simulink model "final"  (R2024a)
settings: Solver=ode23t  StartTime=0.0  StopTime=1  RelTol=1e-6
model workspace (MAT data in the model file):
  Ts = 0.10201388834
undefined symbols (not defined in the file or in its folder): DiscIntNeverNeededParam, Ion, Lithium
libraries: spsIGBTDiodeLib x13, slpidlib x9, spsSeriesRLCBranchLib x7, spsCurrentMeasurementLib x6, spsThreePhaseSeriesRLCBranchLib x6, spsThreePhaseVIMeasurementLib x5, spsAlphaBetaZerotodq0Lib x4, spsGroundLib x3, spsPower3phInstantaneousLib x3, spsMosfetLib x2, simulink x2, spsdq0toabcLib x2
(part 2 of 3)

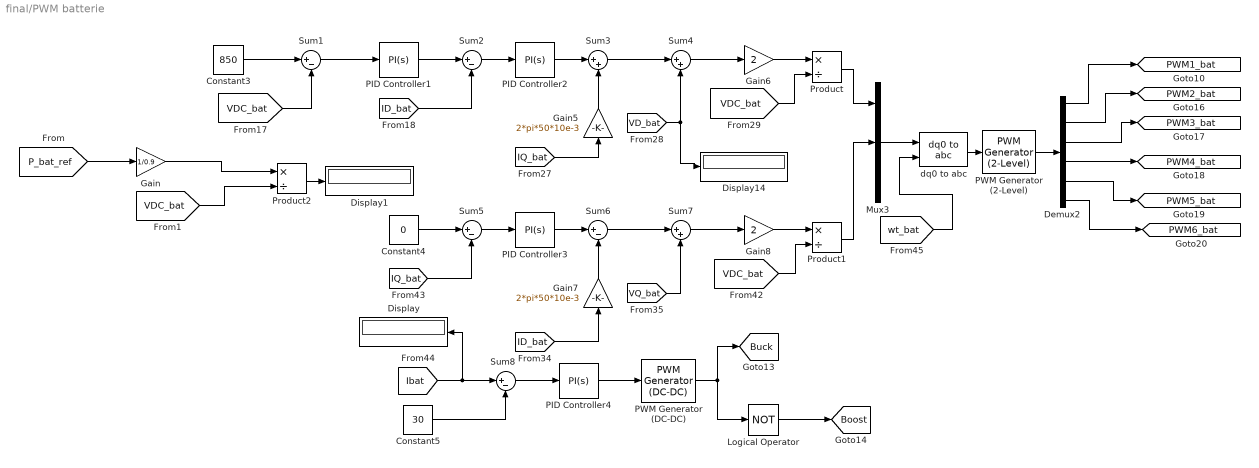
== system final/PWM batterie ==
  Constant3 : Constant  Value=850
  Constant4 : Constant  Value=0
  Constant5 : Constant  Value=30
  Demux2 : Demux  Outputs=6
  Display : Display
  Display1 : Display
  Display14 : Display
  Gain : Gain  Gain=1/0.9
  Gain5 : Gain  Gain=2*pi*50*10e-3
  Gain6 : Gain  Gain=2
  Gain7 : Gain  Gain=2*pi*50*10e-3
  Gain8 : Gain  Gain=2
  Logical Operator : Logic  Operator=NOT  AllPortsSameDT=off  OutDataTypeStr=boolean
  Mux3 : Mux  Inputs=3
  PID Controller1 : slpidlib/PID Controller  Controller=PI  Form=Parallel  TimeDomain=Continuous-time  UseExternalTs=off  SampleTime=-1  IntegratorMethod=Forward Euler  FilterMethod=Forward Euler  ControllerParametersSource=internal  P=0.5  I=5  UseKiTs=off  D=0  UseExternalDerivativeSource=off  N=100  UseFilter=on  TunerSelectOption=Transfer Function Based (PID Tuner App)  InitialConditionSource=internal  InitialConditionForIntegrator=0  InitialConditionForFilter=0  DifferentiatorICPrevScaledInput=0  ExternalReset=none  TrackingMode=off  Kt=1  LimitOutput=off  SatLimitsSource=internal  UpperSaturationLimit=inf  LowerSaturationLimit=-inf  LinearizeAsGain=on  AntiWindupMode=none  Kb=1  LimitIntegrator=off  UpperIntegratorSaturationLimit=inf  LowerIntegratorSaturationLimit=-inf  POutMin=[]  POutMax=[]  IOutMin=[]  IOutMax=[]  DOutMin=[]  DOutMax=[]  NOutMin=[]  NOutMax=[]  SumOutMin=[]  SumOutMax=[]  SaturationOutMin=[]  SaturationOutMax=[]  PParamMin=[]  PParamMax=[]  IParamMin=[]  IParamMax=[]  DParamMin=[]  DParamMax=[]  NParamMin=[]  NParamMax=[]  KbParamMin=[]  KbParamMax=[]  KtParamMin=[]  KtParamMax=[]  KbOutMin=[]  KbOutMax=[]  KtOutMin=[]  KtOutMax=[]  IntegratorOutMin=[]  IntegratorOutMax=[]  FilterOutMin=[]  FilterOutMax=[]  SumI1OutMin=[]  SumI1OutMax=[]  SumI2OutMin=[]  SumI2OutMax=[]  SumI3OutMin=[]  SumI3OutMax=[]  SumI4OutMin=[]  SumI4OutMax=[]  SumDOutMin=[]  SumDOutMax=[]  DifferentiatorOutMin=[]  DifferentiatorOutMax=[]  FilterDiffOutCoefMin=[]  FilterDiffOutCoefMax=[]  ReciprocalOutMin=[]  ReciprocalOutMax=[]  SumDenOutMin=[]  SumDenOutMax=[]  SumNumOutMin=[]  SumNumOutMax=[]  DivideOutMin=[]  DivideOutMax=[]  UdiffTsProdOutMin=[]  UdiffTsProdOutMax=[]  NTsProdOutMin=[]  NTsProdOutMax=[]  UintegralTsProdOutMin=[]  UintegralTsProdOutMax=[]  UngainTsProdOutMin=[]  UngainTsProdOutMax=[]  ClampingZeroOutDataTypeStr=Inherit: Inherit via back propagation  ClampingZeroOutMin=[]  ClampingZeroOutMax=[]  FilterDenConstantOutDataTypeStr=Inherit: Inherit via back propagation  FilterDenConstantOutMin=[]  FilterDenConstantOutMax=[]  PCopyOutDataTypeStr=Inherit: Inherit via back propagation  PCopyOutMin=[]  PCopyOutMax=[]  NCopyOutDataTypeStr=Inherit: Inherit via back propagation  NCopyOutMin=[]  NCopyOutMax=[]  IntegratorContinuousStateAttributes=''  IntegratorStateMustResolveToSignalObject=off  IntegratorRTWStateStorageClass=Auto  FilterContinuousStateAttributes=''  FilterStateMustResolveToSignalObject=off  FilterRTWStateStorageClass=Auto  ParallelPVariant=InternalParameters  IdealPVariant=Disabled  IVariant=InternalParameters  DVariant=Disabled  IntegratorVariant=Continuous  SatVariant=Disabled  AWVariant=Passthrough  PCopyVariant=Disabled  TRVariant=Disabled  FdbkBlocksVariant=Forward  IdealPFdbkVariant=Disabled  SatFdbkVariant=Disabled  DerivativeFilterVariant=Disabled  NVariant=Disabled  NCopyVariant=Disabled_SignalSpec  FilterICVariant=Disabled  IntegratorICVariant=InternalICs  ExternalResetVariant=Disabled  TRSumVariant=Passthrough  SumFdbkVariant=Disabled  SumVariant=Sum_PI  TsampFilterVariant=InternalTs  TsampNgainVariant=Passthrough  TsampIntegralVariant=Disabled_SignalSpec  ExternalSaturationOutDataTypeStr=Inherit: Same as second input  DerivativeSourceVariant=Disabled
  PID Controller2 : slpidlib/PID Controller  Controller=PI  Form=Parallel  TimeDomain=Continuous-time  UseExternalTs=off  SampleTime=-1  IntegratorMethod=Forward Euler  FilterMethod=Forward Euler  ControllerParametersSource=internal  P=25  I=500  UseKiTs=off  D=0  UseExternalDerivativeSource=off  N=100  UseFilter=on  TunerSelectOption=Transfer Function Based (PID Tuner App)  InitialConditionSource=internal  InitialConditionForIntegrator=0  InitialConditionForFilter=0  DifferentiatorICPrevScaledInput=0  ExternalReset=none  TrackingMode=off  Kt=1  LimitOutput=off  SatLimitsSource=internal  UpperSaturationLimit=inf  LowerSaturationLimit=-inf  LinearizeAsGain=on  AntiWindupMode=none  Kb=1  LimitIntegrator=off  UpperIntegratorSaturationLimit=inf  LowerIntegratorSaturationLimit=-inf  POutMin=[]  POutMax=[]  IOutMin=[]  IOutMax=[]  DOutMin=[]  DOutMax=[]  NOutMin=[]  NOutMax=[]  SumOutMin=[]  SumOutMax=[]  SaturationOutMin=[]  SaturationOutMax=[]  PParamMin=[]  PParamMax=[]  IParamMin=[]  IParamMax=[]  DParamMin=[]  DParamMax=[]  NParamMin=[]  NParamMax=[]  KbParamMin=[]  KbParamMax=[]  KtParamMin=[]  KtParamMax=[]  KbOutMin=[]  KbOutMax=[]  KtOutMin=[]  KtOutMax=[]  IntegratorOutMin=[]  IntegratorOutMax=[]  FilterOutMin=[]  FilterOutMax=[]  SumI1OutMin=[]  SumI1OutMax=[]  SumI2OutMin=[]  SumI2OutMax=[]  SumI3OutMin=[]  SumI3OutMax=[]  SumI4OutMin=[]  SumI4OutMax=[]  SumDOutMin=[]  SumDOutMax=[]  DifferentiatorOutMin=[]  DifferentiatorOutMax=[]  FilterDiffOutCoefMin=[]  FilterDiffOutCoefMax=[]  ReciprocalOutMin=[]  ReciprocalOutMax=[]  SumDenOutMin=[]  SumDenOutMax=[]  SumNumOutMin=[]  SumNumOutMax=[]  DivideOutMin=[]  DivideOutMax=[]  UdiffTsProdOutMin=[]  UdiffTsProdOutMax=[]  NTsProdOutMin=[]  NTsProdOutMax=[]  UintegralTsProdOutMin=[]  UintegralTsProdOutMax=[]  UngainTsProdOutMin=[]  UngainTsProdOutMax=[]  ClampingZeroOutDataTypeStr=Inherit: Inherit via back propagation  ClampingZeroOutMin=[]  ClampingZeroOutMax=[]  FilterDenConstantOutDataTypeStr=Inherit: Inherit via back propagation  FilterDenConstantOutMin=[]  FilterDenConstantOutMax=[]  PCopyOutDataTypeStr=Inherit: Inherit via back propagation  PCopyOutMin=[]  PCopyOutMax=[]  NCopyOutDataTypeStr=Inherit: Inherit via back propagation  NCopyOutMin=[]  NCopyOutMax=[]  IntegratorContinuousStateAttributes=''  IntegratorStateMustResolveToSignalObject=off  IntegratorRTWStateStorageClass=Auto  FilterContinuousStateAttributes=''  FilterStateMustResolveToSignalObject=off  FilterRTWStateStorageClass=Auto  ParallelPVariant=InternalParameters  IdealPVariant=Disabled  IVariant=InternalParameters  DVariant=Disabled  IntegratorVariant=Continuous  SatVariant=Disabled  AWVariant=Passthrough  PCopyVariant=Disabled  TRVariant=Disabled  FdbkBlocksVariant=Forward  IdealPFdbkVariant=Disabled  SatFdbkVariant=Disabled  DerivativeFilterVariant=Disabled  NVariant=Disabled  NCopyVariant=Disabled_SignalSpec  FilterICVariant=Disabled  IntegratorICVariant=InternalICs  ExternalResetVariant=Disabled  TRSumVariant=Passthrough  SumFdbkVariant=Disabled  SumVariant=Sum_PI  TsampFilterVariant=InternalTs  TsampNgainVariant=Passthrough  TsampIntegralVariant=Disabled_SignalSpec  ExternalSaturationOutDataTypeStr=Inherit: Same as second input  DerivativeSourceVariant=Disabled
  PID Controller3 : slpidlib/PID Controller  Controller=PI  Form=Parallel  TimeDomain=Continuous-time  UseExternalTs=off  SampleTime=-1  IntegratorMethod=Forward Euler  FilterMethod=Forward Euler  ControllerParametersSource=internal  P=25  I=500  UseKiTs=off  D=0  UseExternalDerivativeSource=off  N=100  UseFilter=on  TunerSelectOption=Transfer Function Based (PID Tuner App)  InitialConditionSource=internal  InitialConditionForIntegrator=0  InitialConditionForFilter=0  DifferentiatorICPrevScaledInput=0  ExternalReset=none  TrackingMode=off  Kt=1  LimitOutput=off  SatLimitsSource=internal  UpperSaturationLimit=inf  LowerSaturationLimit=-inf  LinearizeAsGain=on  AntiWindupMode=none  Kb=1  LimitIntegrator=off  UpperIntegratorSaturationLimit=inf  LowerIntegratorSaturationLimit=-inf  POutMin=[]  POutMax=[]  IOutMin=[]  IOutMax=[]  DOutMin=[]  DOutMax=[]  NOutMin=[]  NOutMax=[]  SumOutMin=[]  SumOutMax=[]  SaturationOutMin=[]  SaturationOutMax=[]  PParamMin=[]  PParamMax=[]  IParamMin=[]  IParamMax=[]  DParamMin=[]  DParamMax=[]  NParamMin=[]  NParamMax=[]  KbParamMin=[]  KbParamMax=[]  KtParamMin=[]  KtParamMax=[]  KbOutMin=[]  KbOutMax=[]  KtOutMin=[]  KtOutMax=[]  IntegratorOutMin=[]  IntegratorOutMax=[]  FilterOutMin=[]  FilterOutMax=[]  SumI1OutMin=[]  SumI1OutMax=[]  SumI2OutMin=[]  SumI2OutMax=[]  SumI3OutMin=[]  SumI3OutMax=[]  SumI4OutMin=[]  SumI4OutMax=[]  SumDOutMin=[]  SumDOutMax=[]  DifferentiatorOutMin=[]  DifferentiatorOutMax=[]  FilterDiffOutCoefMin=[]  FilterDiffOutCoefMax=[]  ReciprocalOutMin=[]  ReciprocalOutMax=[]  SumDenOutMin=[]  SumDenOutMax=[]  SumNumOutMin=[]  SumNumOutMax=[]  DivideOutMin=[]  DivideOutMax=[]  UdiffTsProdOutMin=[]  UdiffTsProdOutMax=[]  NTsProdOutMin=[]  NTsProdOutMax=[]  UintegralTsProdOutMin=[]  UintegralTsProdOutMax=[]  UngainTsProdOutMin=[]  UngainTsProdOutMax=[]  ClampingZeroOutDataTypeStr=Inherit: Inherit via back propagation  ClampingZeroOutMin=[]  ClampingZeroOutMax=[]  FilterDenConstantOutDataTypeStr=Inherit: Inherit via back propagation  FilterDenConstantOutMin=[]  FilterDenConstantOutMax=[]  PCopyOutDataTypeStr=Inherit: Inherit via back propagation  PCopyOutMin=[]  PCopyOutMax=[]  NCopyOutDataTypeStr=Inherit: Inherit via back propagation  NCopyOutMin=[]  NCopyOutMax=[]  IntegratorContinuousStateAttributes=''  IntegratorStateMustResolveToSignalObject=off  IntegratorRTWStateStorageClass=Auto  FilterContinuousStateAttributes=''  FilterStateMustResolveToSignalObject=off  FilterRTWStateStorageClass=Auto  ParallelPVariant=InternalParameters  IdealPVariant=Disabled  IVariant=InternalParameters  DVariant=Disabled  IntegratorVariant=Continuous  SatVariant=Disabled  AWVariant=Passthrough  PCopyVariant=Disabled  TRVariant=Disabled  FdbkBlocksVariant=Forward  IdealPFdbkVariant=Disabled  SatFdbkVariant=Disabled  DerivativeFilterVariant=Disabled  NVariant=Disabled  NCopyVariant=Disabled_SignalSpec  FilterICVariant=Disabled  IntegratorICVariant=InternalICs  ExternalResetVariant=Disabled  TRSumVariant=Passthrough  SumFdbkVariant=Disabled  SumVariant=Sum_PI  TsampFilterVariant=InternalTs  TsampNgainVariant=Passthrough  TsampIntegralVariant=Disabled_SignalSpec  ExternalSaturationOutDataTypeStr=Inherit: Same as second input  DerivativeSourceVariant=Disabled
  PID Controller4 : slpidlib/PID Controller  Controller=PI  Form=Parallel  TimeDomain=Continuous-time  UseExternalTs=off  SampleTime=-1  IntegratorMethod=Forward Euler  FilterMethod=Forward Euler  ControllerParametersSource=internal  P=0.005  I=10  UseKiTs=off  D=0  UseExternalDerivativeSource=off  N=100  UseFilter=on  TunerSelectOption=Transfer Function Based (PID Tuner App)  InitialConditionSource=internal  InitialConditionForIntegrator=0  InitialConditionForFilter=0  DifferentiatorICPrevScaledInput=0  ExternalReset=none  TrackingMode=off  Kt=1  LimitOutput=on  SatLimitsSource=internal  UpperSaturationLimit=0.95  LowerSaturationLimit=0  LinearizeAsGain=on  AntiWindupMode=none  Kb=1  LimitIntegrator=off  UpperIntegratorSaturationLimit=inf  LowerIntegratorSaturationLimit=-inf  POutMin=[]  POutMax=[]  IOutMin=[]  IOutMax=[]  DOutMin=[]  DOutMax=[]  NOutMin=[]  NOutMax=[]  SumOutMin=[]  SumOutMax=[]  SaturationOutMin=[]  SaturationOutMax=[]  PParamMin=[]  PParamMax=[]  IParamMin=[]  IParamMax=[]  DParamMin=[]  DParamMax=[]  NParamMin=[]  NParamMax=[]  KbParamMin=[]  KbParamMax=[]  KtParamMin=[]  KtParamMax=[]  KbOutMin=[]  KbOutMax=[]  KtOutMin=[]  KtOutMax=[]  IntegratorOutMin=[]  IntegratorOutMax=[]  FilterOutMin=[]  FilterOutMax=[]  SumI1OutMin=[]  SumI1OutMax=[]  SumI2OutMin=[]  SumI2OutMax=[]  SumI3OutMin=[]  SumI3OutMax=[]  SumI4OutMin=[]  SumI4OutMax=[]  SumDOutMin=[]  SumDOutMax=[]  DifferentiatorOutMin=[]  DifferentiatorOutMax=[]  FilterDiffOutCoefMin=[]  FilterDiffOutCoefMax=[]  ReciprocalOutMin=[]  ReciprocalOutMax=[]  SumDenOutMin=[]  SumDenOutMax=[]  SumNumOutMin=[]  SumNumOutMax=[]  DivideOutMin=[]  DivideOutMax=[]  UdiffTsProdOutMin=[]  UdiffTsProdOutMax=[]  NTsProdOutMin=[]  NTsProdOutMax=[]  UintegralTsProdOutMin=[]  UintegralTsProdOutMax=[]  UngainTsProdOutMin=[]  UngainTsProdOutMax=[]  ClampingZeroOutDataTypeStr=Inherit: Inherit via back propagation  ClampingZeroOutMin=[]  ClampingZeroOutMax=[]  FilterDenConstantOutDataTypeStr=Inherit: Inherit via back propagation  FilterDenConstantOutMin=[]  FilterDenConstantOutMax=[]  PCopyOutDataTypeStr=Inherit: Inherit via back propagation  PCopyOutMin=[]  PCopyOutMax=[]  NCopyOutDataTypeStr=Inherit: Inherit via back propagation  NCopyOutMin=[]  NCopyOutMax=[]  IntegratorContinuousStateAttributes=''  IntegratorStateMustResolveToSignalObject=off  IntegratorRTWStateStorageClass=Auto  FilterContinuousStateAttributes=''  FilterStateMustResolveToSignalObject=off  FilterRTWStateStorageClass=Auto  ParallelPVariant=InternalParameters  IdealPVariant=Disabled  IVariant=InternalParameters  DVariant=Disabled  IntegratorVariant=Continuous  SatVariant=Enabled  AWVariant=Passthrough  PCopyVariant=Disabled  TRVariant=Disabled  FdbkBlocksVariant=Forward  IdealPFdbkVariant=Disabled  SatFdbkVariant=Disabled  DerivativeFilterVariant=Disabled  NVariant=Disabled  NCopyVariant=Disabled_SignalSpec  FilterICVariant=Disabled  IntegratorICVariant=InternalICs  ExternalResetVariant=Disabled  TRSumVariant=Passthrough  SumFdbkVariant=Disabled  SumVariant=Sum_PI  TsampFilterVariant=InternalTs  TsampNgainVariant=Passthrough  TsampIntegralVariant=Disabled_SignalSpec  ExternalSaturationOutDataTypeStr=Inherit: Same as second input  DerivativeSourceVariant=Disabled
  PWM Generator (2-Level) : spsPWMGenerator2LevelLib/PWM Generator (2-Level)  ModulatorType=Three-phase bridge (6 pulses)  ModulatorMode=Unsynchronized  Fc=10000  Pc=90  nF=27  MinMax="[ -1  1 ]"  SamplingTechnique=Natural  ModulatingSignals=off  m=0.8  Freq=60  Phase=0  Ts=0  ShowCarrierOutport=off
  PWM Generator (DC-DC) : spsPWMGeneratorDCDCLib/PWM Generator (DC-DC)  Fsw=10000  Ts=0
  Product : Product  Inputs=*/
  Product1 : Product  Inputs=*/
  Product2 : Product  Inputs=*/
  Sum{1..2,5..6,8} (5 alike) : Sum  Inputs=|+-
  Sum3 : Sum  Inputs=|++
  Sum4 : Sum  Inputs=|++
  Sum7 : Sum  Inputs=|++
  dq0 to abc : spsdq0toabcLib/dq0 to abc  Alignment=90 degrees behind phase A axis
  tag scope: Boost=global, Buck=global, PWM1_bat=global, PWM2_bat=global, PWM3_bat=global, PWM4_bat=global, PWM5_bat=global, PWM6_bat=global
  wires:
  dq0 to abc/1 -> PWM Generator (2-Level)/1
  Constant3/1 -> Sum1/1
  [Ibat] -> Display/1, Sum8/1
  [VDC_bat] -> Product/2
  Logical Operator/1 -> [Boost]
  [VQ_bat] -> Sum7/2
  [IQ_bat] -> Gain5/1
  Constant4/1 -> Sum5/1
  [IQ_bat] -> Sum5/2
  [ID_bat] -> Sum2/2
  Gain7/1 -> Sum6/2
  Mux3/1 -> dq0 to abc/1
  [VD_bat] -> Display14/1, Sum4/2
  Sum6/1 -> Sum7/1
  Sum8/1 -> PID Controller4/1
  PWM Generator (DC-DC)/1 -> [Buck], Logical Operator/1
  [wt_bat] -> dq0 to abc/2
  Gain8/1 -> Product1/1
  Demux2/1 -> [PWM1_bat]
  Product1/1 -> Mux3/2
  Demux2/5 -> [PWM5_bat]
  Sum7/1 -> Gain8/1
  [ID_bat] -> Gain7/1
  Demux2/4 -> [PWM4_bat]
  PID Controller4/1 -> PWM Generator (DC-DC)/1
  Sum2/1 -> PID Controller2/1
  Gain6/1 -> Product/1
  Gain5/1 -> Sum3/2
  Sum5/1 -> PID Controller3/1
  Sum3/1 -> Sum4/1
  [VDC_bat] -> Product1/2
  Sum1/1 -> PID Controller1/1
  Demux2/6 -> [PWM6_bat]
  PID Controller3/1 -> Sum6/1
  PWM Generator (2-Level)/1 -> Demux2/1
  Product/1 -> Mux3/1
  Demux2/2 -> [PWM2_bat]
  PID Controller1/1 -> Sum2/1
  Constant5/1 -> Sum8/2
  Demux2/3 -> [PWM3_bat]
  Sum4/1 -> Gain6/1
  PID Controller2/1 -> Sum3/1
  [VDC_bat] -> Sum1/2
  [P_bat_ref] -> Gain/1
  Gain/1 -> Product2/1
  [VDC_bat] -> Product2/2
  Product2/1 -> Display1/1

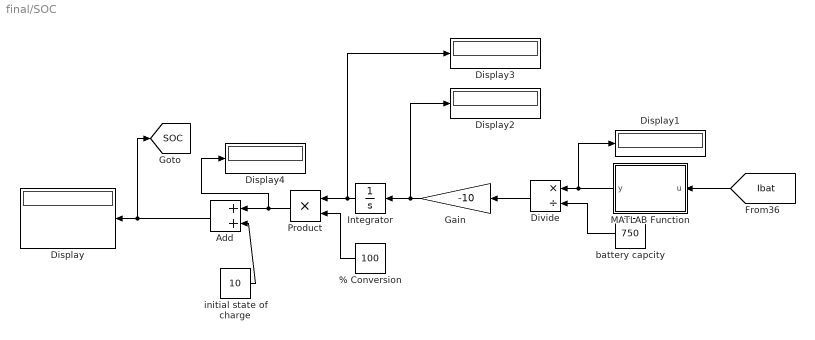
== system final/SOC  ==
  "% Conversion " : Constant  Value=100
  Add : Sum
  Display{,1..4} (5 alike) : Display
  Divide : Product  Inputs=*/
  Gain : Gain  Gain=-10
  Integrator : Integrator
  MATLAB Function : MATLAB Function  TreatAsAtomicUnit=on
  Product : Product
  battery capcity : Constant  Value=750
  initial state of charge : Constant  Value=10
  tag scope: SOC=global
  wires:
  MATLAB Function/1(y) -> Display1/1, Divide/1
  Product/1 -> Display4/1, Add/1
  Add/1 -> [SOC], Display/1
  "% Conversion "/1 -> Product/2
  initial state of charge/1 -> Add/2
  battery capcity/1 -> Divide/2
  Divide/1 -> Gain/1
  Integrator/1 -> Display3/1, Product/1
  Gain/1 -> Display2/1, Integrator/1
  [Ibat] -> MATLAB Function/1(u)

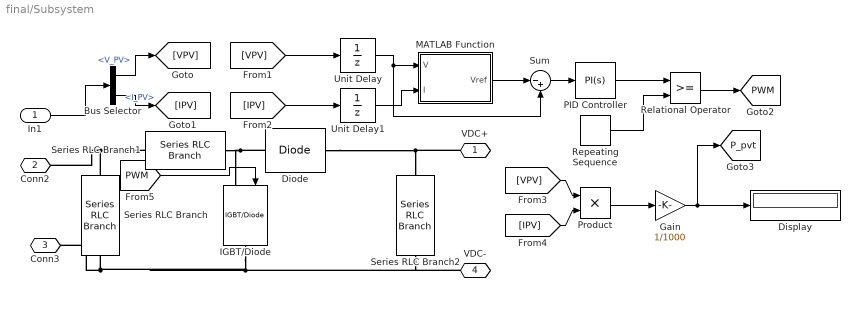
== system final/Subsystem ==
  In1 : Inport
  Bus Selector : BusSelector  OutputSignals=V_PV,I_PV
  Diode : spsDiodeLib/Diode  Ron=0.001  Lon=0  Vf=0.8  IC=0  UseSnubber=0  Rs=500  Cs=250e-9  Measurements=off
  Display : Display
  Gain : Gain  Gain=1/1000
  IGBT/Diode : spsIGBTDiodeLib/IGBT//Diode  Ron=1e-3  Rs=1e5  Cs=inf  Measurements=off
  MATLAB Function : MATLAB Function  TreatAsAtomicUnit=on
  PID Controller : slpidlib/PID Controller  Controller=PI  Form=Parallel  TimeDomain=Continuous-time  UseExternalTs=off  SampleTime=-1  IntegratorMethod=Forward Euler  FilterMethod=Forward Euler  ControllerParametersSource=internal  P=0.005  I=0.001  UseKiTs=off  D=0  UseExternalDerivativeSource=off  N=100  UseFilter=on  TunerSelectOption=Transfer Function Based (PID Tuner App)  InitialConditionSource=internal  InitialConditionForIntegrator=0  InitialConditionForFilter=0  DifferentiatorICPrevScaledInput=0  ExternalReset=none  TrackingMode=off  Kt=1  LimitOutput=on  SatLimitsSource=internal  UpperSaturationLimit=0.95  LowerSaturationLimit=0  LinearizeAsGain=on  AntiWindupMode=none  Kb=1  LimitIntegrator=off  UpperIntegratorSaturationLimit=inf  LowerIntegratorSaturationLimit=-inf  POutMin=[]  POutMax=[]  IOutMin=[]  IOutMax=[]  DOutMin=[]  DOutMax=[]  NOutMin=[]  NOutMax=[]  SumOutMin=[]  SumOutMax=[]  SaturationOutMin=[]  SaturationOutMax=[]  PParamMin=[]  PParamMax=[]  IParamMin=[]  IParamMax=[]  DParamMin=[]  DParamMax=[]  NParamMin=[]  NParamMax=[]  KbParamMin=[]  KbParamMax=[]  KtParamMin=[]  KtParamMax=[]  KbOutMin=[]  KbOutMax=[]  KtOutMin=[]  KtOutMax=[]  IntegratorOutMin=[]  IntegratorOutMax=[]  FilterOutMin=[]  FilterOutMax=[]  SumI1OutMin=[]  SumI1OutMax=[]  SumI2OutMin=[]  SumI2OutMax=[]  SumI3OutMin=[]  SumI3OutMax=[]  SumI4OutMin=[]  SumI4OutMax=[]  SumDOutMin=[]  SumDOutMax=[]  DifferentiatorOutMin=[]  DifferentiatorOutMax=[]  FilterDiffOutCoefMin=[]  FilterDiffOutCoefMax=[]  ReciprocalOutMin=[]  ReciprocalOutMax=[]  SumDenOutMin=[]  SumDenOutMax=[]  SumNumOutMin=[]  SumNumOutMax=[]  DivideOutMin=[]  DivideOutMax=[]  UdiffTsProdOutMin=[]  UdiffTsProdOutMax=[]  NTsProdOutMin=[]  NTsProdOutMax=[]  UintegralTsProdOutMin=[]  UintegralTsProdOutMax=[]  UngainTsProdOutMin=[]  UngainTsProdOutMax=[]  ClampingZeroOutDataTypeStr=Inherit: Inherit via back propagation  ClampingZeroOutMin=[]  ClampingZeroOutMax=[]  FilterDenConstantOutDataTypeStr=Inherit: Inherit via back propagation  FilterDenConstantOutMin=[]  FilterDenConstantOutMax=[]  PCopyOutDataTypeStr=Inherit: Inherit via back propagation  PCopyOutMin=[]  PCopyOutMax=[]  NCopyOutDataTypeStr=Inherit: Inherit via back propagation  NCopyOutMin=[]  NCopyOutMax=[]  IntegratorContinuousStateAttributes=''  IntegratorStateMustResolveToSignalObject=off  IntegratorRTWStateStorageClass=Auto  FilterContinuousStateAttributes=''  FilterStateMustResolveToSignalObject=off  FilterRTWStateStorageClass=Auto  ParallelPVariant=InternalParameters  IdealPVariant=Disabled  IVariant=InternalParameters  DVariant=Disabled  IntegratorVariant=Continuous  SatVariant=Enabled  AWVariant=Passthrough  PCopyVariant=Disabled  TRVariant=Disabled  FdbkBlocksVariant=Forward  IdealPFdbkVariant=Disabled  SatFdbkVariant=Disabled  DerivativeFilterVariant=Disabled  NVariant=Disabled  NCopyVariant=Disabled_SignalSpec  FilterICVariant=Disabled  IntegratorICVariant=InternalICs  ExternalResetVariant=Disabled  TRSumVariant=Passthrough  SumFdbkVariant=Disabled  SumVariant=Sum_PI  TsampFilterVariant=InternalTs  TsampNgainVariant=Passthrough  TsampIntegralVariant=Disabled_SignalSpec  ExternalSaturationOutDataTypeStr=Inherit: Same as second input  DerivativeSourceVariant=Disabled
  Product : Product
  Relational Operator : RelationalOperator  OutDataTypeStr=boolean  RndMeth=Simplest  InputSameDT=off
  Repeating Sequence : simulink/Sources/Repeating Sequence  rep_seq_t=[0 0.0002]  rep_seq_y=[0 1]
  Series RLC Branch : spsSeriesRLCBranchLib/Series RLC Branch  LConnTagsString=__new0  RConnTagsString=__new0  BranchType=RC  Resistance=1e-3  Inductance=1e-3  SetiL0=off  InitialCurrent=0  Capacitance=1000e-3  Setx0=off  InitialVoltage=600  Measurements=None
  Series RLC Branch1 : spsSeriesRLCBranchLib/Series RLC Branch  LConnTagsString=__new0  RConnTagsString=__new0  BranchType=L  Resistance=1e-3  Inductance=1.45e-3  SetiL0=off  InitialCurrent=0  Capacitance=1000e-6  Setx0=off  InitialVoltage=0  Measurements=None
  Series RLC Branch2 : spsSeriesRLCBranchLib/Series RLC Branch  LConnTagsString=__new0  RConnTagsString=__new0  BranchType=C  Resistance=1e-3  Inductance=1.45e-3  SetiL0=off  InitialCurrent=0  Capacitance=3227e-6  Setx0=on  InitialVoltage=330  Measurements=None
  Sum : Sum  Inputs=|-+
  Unit Delay : UnitDelay  SampleTime=1e-4  HasFrameUpgradeWarning=on
  Unit Delay1 : UnitDelay  SampleTime=1e-4  HasFrameUpgradeWarning=on
  VDC+ : PMIOPort  Side=Right
  Conn2 : PMIOPort  Port=2  Side=Left
  Conn3 : PMIOPort  Port=3  Side=Left
  VDC- : PMIOPort  Port=4  Side=Right
  tag scope: PWM=global, P_pvt=global
  wires:
  [IPV] -> Unit Delay1/1
  Bus Selector/2 -> [IPV]  "<I_PV>"
  Relational Operator/1 -> [PWM]
  MATLAB Function/1(Vref) -> Sum/1
  Bus Selector/1 -> [VPV]  "<V_PV>"
  [PWM] -> IGBT/Diode/1
  Sum/1 -> PID Controller/1
  [VPV] -> Unit Delay/1
  Unit Delay1/1 -> MATLAB Function/2(I)
  Unit Delay/1 -> MATLAB Function/1(V), Sum/2
  PID Controller/1 -> Relational Operator/1
  In1/1 -> Bus Selector/1
  Repeating Sequence/1 -> Relational Operator/2
  Gain/1 -> [P_pvt], Display/1
  Product/1 -> Gain/1
  [VPV] -> Product/1
  [IPV] -> Product/2
  connections:
  Series RLC Branch/LConn1 -- Series RLC Branch1/RConn1 -- Conn2/RConn1
  Series RLC Branch1/LConn1 -- IGBT/Diode/LConn1 -- Diode/LConn1
  VDC+/RConn1 -- Series RLC Branch2/LConn1 -- Diode/RConn1
  Series RLC Branch/RConn1 -- VDC-/RConn1 -- Series RLC Branch2/RConn1 -- IGBT/Diode/RConn1 -- Conn3/RConn1

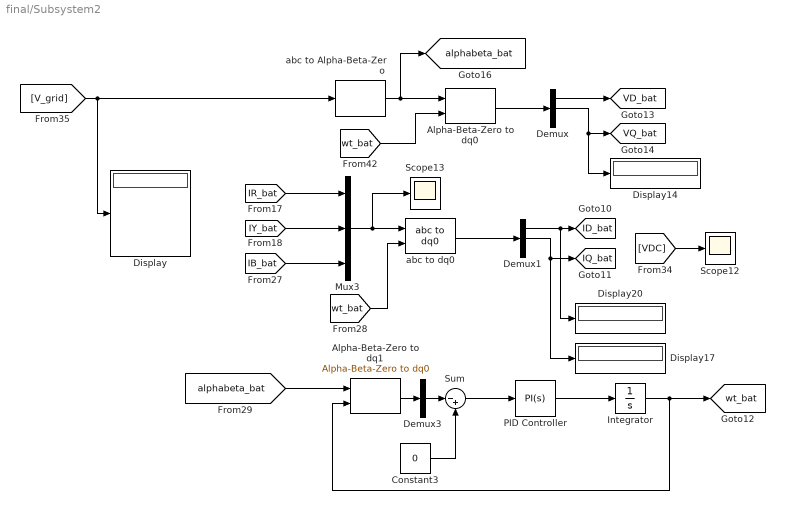
== system final/Subsystem2 ==
  Alpha-Beta-Zero to dq0 : spsAlphaBetaZerotodq0Lib/Alpha-Beta-Zero to dq0  Alignment=90 degrees behind phase A axis
  Alpha-Beta-Zero to dq1 : spsAlphaBetaZerotodq0Lib/Alpha-Beta-Zero to dq0  Alignment=90 degrees behind phase A axis
  Constant3 : Constant  Value=0
  Demux : Demux  Outputs=3
  Demux1 : Demux  Outputs=3
  Demux3 : Demux  Outputs=3
  Display{,14,17,20} (4 alike) : Display
  Integrator : Integrator
  Mux3 : Mux  Inputs=3
  PID Controller : slpidlib/PID Controller  Controller=PI  Form=Parallel  TimeDomain=Continuous-time  UseExternalTs=off  SampleTime=-1  IntegratorMethod=Forward Euler  FilterMethod=Forward Euler  ControllerParametersSource=internal  P=10  I=50000  UseKiTs=off  D=0  UseExternalDerivativeSource=off  N=100  UseFilter=on  TunerSelectOption=Transfer Function Based (PID Tuner App)  InitialConditionSource=internal  InitialConditionForIntegrator=0  InitialConditionForFilter=0  DifferentiatorICPrevScaledInput=0  ExternalReset=none  TrackingMode=off  Kt=1  LimitOutput=off  SatLimitsSource=internal  UpperSaturationLimit=inf  LowerSaturationLimit=-inf  LinearizeAsGain=on  AntiWindupMode=none  Kb=1  LimitIntegrator=off  UpperIntegratorSaturationLimit=inf  LowerIntegratorSaturationLimit=-inf  POutMin=[]  POutMax=[]  IOutMin=[]  IOutMax=[]  DOutMin=[]  DOutMax=[]  NOutMin=[]  NOutMax=[]  SumOutMin=[]  SumOutMax=[]  SaturationOutMin=[]  SaturationOutMax=[]  PParamMin=[]  PParamMax=[]  IParamMin=[]  IParamMax=[]  DParamMin=[]  DParamMax=[]  NParamMin=[]  NParamMax=[]  KbParamMin=[]  KbParamMax=[]  KtParamMin=[]  KtParamMax=[]  KbOutMin=[]  KbOutMax=[]  KtOutMin=[]  KtOutMax=[]  IntegratorOutMin=[]  IntegratorOutMax=[]  FilterOutMin=[]  FilterOutMax=[]  SumI1OutMin=[]  SumI1OutMax=[]  SumI2OutMin=[]  SumI2OutMax=[]  SumI3OutMin=[]  SumI3OutMax=[]  SumI4OutMin=[]  SumI4OutMax=[]  SumDOutMin=[]  SumDOutMax=[]  DifferentiatorOutMin=[]  DifferentiatorOutMax=[]  FilterDiffOutCoefMin=[]  FilterDiffOutCoefMax=[]  ReciprocalOutMin=[]  ReciprocalOutMax=[]  SumDenOutMin=[]  SumDenOutMax=[]  SumNumOutMin=[]  SumNumOutMax=[]  DivideOutMin=[]  DivideOutMax=[]  UdiffTsProdOutMin=[]  UdiffTsProdOutMax=[]  NTsProdOutMin=[]  NTsProdOutMax=[]  UintegralTsProdOutMin=[]  UintegralTsProdOutMax=[]  UngainTsProdOutMin=[]  UngainTsProdOutMax=[]  ClampingZeroOutDataTypeStr=Inherit: Inherit via back propagation  ClampingZeroOutMin=[]  ClampingZeroOutMax=[]  FilterDenConstantOutDataTypeStr=Inherit: Inherit via back propagation  FilterDenConstantOutMin=[]  FilterDenConstantOutMax=[]  PCopyOutDataTypeStr=Inherit: Inherit via back propagation  PCopyOutMin=[]  PCopyOutMax=[]  NCopyOutDataTypeStr=Inherit: Inherit via back propagation  NCopyOutMin=[]  NCopyOutMax=[]  IntegratorContinuousStateAttributes=''  IntegratorStateMustResolveToSignalObject=off  IntegratorRTWStateStorageClass=Auto  FilterContinuousStateAttributes=''  FilterStateMustResolveToSignalObject=off  FilterRTWStateStorageClass=Auto  ParallelPVariant=InternalParameters  IdealPVariant=Disabled  IVariant=InternalParameters  DVariant=Disabled  IntegratorVariant=Continuous  SatVariant=Disabled  AWVariant=Passthrough  PCopyVariant=Disabled  TRVariant=Disabled  FdbkBlocksVariant=Forward  IdealPFdbkVariant=Disabled  SatFdbkVariant=Disabled  DerivativeFilterVariant=Disabled  NVariant=Disabled  NCopyVariant=Disabled_SignalSpec  FilterICVariant=Disabled  IntegratorICVariant=InternalICs  ExternalResetVariant=Disabled  TRSumVariant=Passthrough  SumFdbkVariant=Disabled  SumVariant=Sum_PI  TsampFilterVariant=InternalTs  TsampNgainVariant=Passthrough  TsampIntegralVariant=Disabled_SignalSpec  ExternalSaturationOutDataTypeStr=Inherit: Same as second input  DerivativeSourceVariant=Disabled
  Scope12 : Scope
  Scope13 : Scope
  Sum : Sum  Inputs=|-+
  abc to Alpha-Beta-Zero : spsabctoAlphaBetaZeroLib/abc to Alpha-Beta-Zero
  abc to dq0 : spsabctodq0Lib/abc to dq0  Alignment=90 degrees behind phase A axis
  tag scope: ID_bat=global, IQ_bat=global, VD_bat=global, VQ_bat=global, alphabeta_bat=global, wt_bat=global
  wires:
  Demux/1 -> [VD_bat]
  Sum/1 -> PID Controller/1
  [alphabeta_bat] -> Alpha-Beta-Zero to dq1/1
  Demux/2 -> Display14/1, [VQ_bat]
  Alpha-Beta-Zero to dq0/1 -> Demux/1
  Integrator/1 -> [wt_bat], Alpha-Beta-Zero to dq1/2
  Demux3/2 -> Sum/1
  Alpha-Beta-Zero to dq1/1 -> Demux3/1
  Demux1/1 -> Display20/1, [ID_bat]
  [wt_bat] -> abc to dq0/2
  [wt_bat] -> Alpha-Beta-Zero to dq0/2
  [IR_bat] -> Mux3/1
  PID Controller/1 -> Integrator/1
  [IY_bat] -> Mux3/2
  [VDC] -> Scope12/1
  [V_grid] -> Display/1, abc to Alpha-Beta-Zero/1
  Mux3/1 -> Scope13/1, abc to dq0/1
  Demux1/2 -> Display17/1, [IQ_bat]
  abc to dq0/1 -> Demux1/1
  Constant3/1 -> Sum/2
  [IB_bat] -> Mux3/3
  abc to Alpha-Beta-Zero/1 -> Alpha-Beta-Zero to dq0/1, [alphabeta_bat]

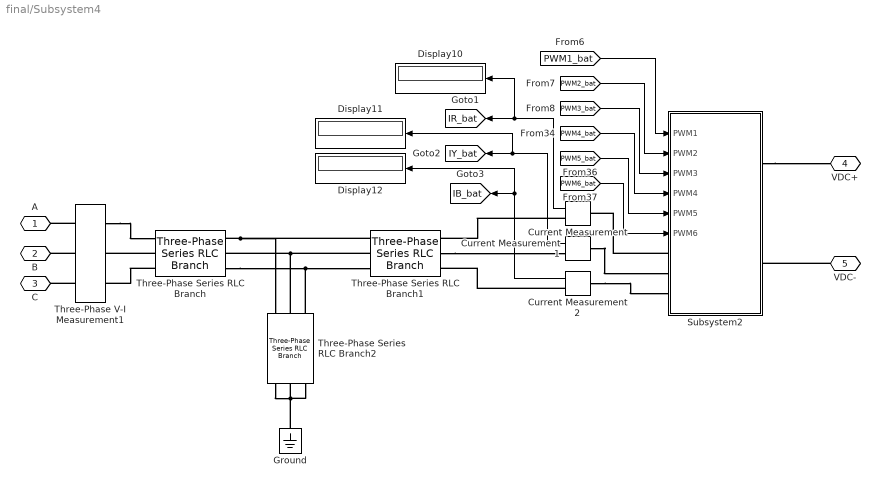
== system final/Subsystem4 ==
  Current Measurement : spsCurrentMeasurementLib/Current Measurement  PhasorSimulation=off  OutputType=Complex  PSBequivalent=0
  Current Measurement1 : spsCurrentMeasurementLib/Current Measurement  PhasorSimulation=off  OutputType=Complex  PSBequivalent=0
  Current Measurement2 : spsCurrentMeasurementLib/Current Measurement  PhasorSimulation=off  OutputType=Complex  PSBequivalent=0
  Display10 : Display
  Display11 : Display
  Display12 : Display
  Ground : spsGroundLib/Ground  LConnTagsString=a
  Subsystem2 : Subsystem
  Three-Phase Series RLC Branch : spsThreePhaseSeriesRLCBranchLib/Three-Phase Series RLC Branch  LConnTagsString=A|B|C  RConnTagsString=A|B|C  BranchType=L  Resistance=1  Inductance=5e-3  Capacitance=1e-6  Measurements=None
  Three-Phase Series RLC Branch1 : spsThreePhaseSeriesRLCBranchLib/Three-Phase Series RLC Branch  LConnTagsString=A|B|C  RConnTagsString=A|B|C  BranchType=L  Resistance=1  Inductance=5e-3  Capacitance=1e-6  Measurements=None
  Three-Phase Series RLC Branch2 : spsThreePhaseSeriesRLCBranchLib/Three-Phase Series RLC Branch  LConnTagsString=A|B|C  RConnTagsString=A|B|C  BranchType=C  Resistance=3291e-4  Inductance=5e-3  Capacitance=30e-6  Measurements=None
  Three-Phase V-I Measurement1 : spsThreePhaseVIMeasurementLib/Three-Phase V-I Measurement  VoltageMeasurement=phase-to-ground  SetLabelV=on  LabelV=Vabc_bat  Vpu=on  VpuLL=off  CurrentMeasurement=yes  SetLabelI=on  LabelI=I_batterie  Ipu=off  Pbase=100e6  Vbase=400  OutputType=Complex  PhasorSimulation=off  PSBequivalent=0
  A : PMIOPort  Side=Left
  B : PMIOPort  Port=2  Side=Left
  C : PMIOPort  Port=3  Side=Left
  VDC+ : PMIOPort  Port=4  Side=Right
  VDC- : PMIOPort  Port=5  Side=Right
  tag scope: IB_bat=global, IR_bat=global, IY_bat=global
  wires:
  [PWM1_bat] -> Subsystem2/1("PWM1 ")
  [PWM6_bat] -> Subsystem2/6(PWM6)
  Current Measurement/1 -> Display10/1, [IR_bat]
  [PWM3_bat] -> Subsystem2/3(PWM3)
  Current Measurement1/1 -> Display11/1, [IY_bat]
  [PWM4_bat] -> Subsystem2/4(PWM4)
  [PWM5_bat] -> Subsystem2/5(PWM5)
  Current Measurement2/1 -> Display12/1, [IB_bat]
  [PWM2_bat] -> Subsystem2/2(PWM2)
  connections:
  Three-Phase V-I Measurement1/LConn1 -- A/RConn1
  Three-Phase Series RLC Branch1/LConn2 -- Three-Phase Series RLC Branch2/LConn2 -- Three-Phase Series RLC Branch/RConn2
  Three-Phase Series RLC Branch/RConn1 -- Three-Phase Series RLC Branch2/LConn1 -- Three-Phase Series RLC Branch1/LConn1
  Current Measurement1/LConn1 -- Subsystem2/LConn2
  Current Measurement2/RConn1 -- Three-Phase Series RLC Branch1/RConn3
  Three-Phase V-I Measurement1/LConn3 -- C/RConn1
  Current Measurement/RConn1 -- Three-Phase Series RLC Branch1/RConn1
  Three-Phase Series RLC Branch1/RConn2 -- Current Measurement1/RConn1
  Subsystem2/RConn1 -- VDC+/RConn1
  Current Measurement2/LConn1 -- Subsystem2/LConn3
  Subsystem2/LConn1 -- Current Measurement/LConn1
  Three-Phase V-I Measurement1/LConn2 -- B/RConn1
  VDC-/RConn1 -- Subsystem2/RConn2
  Three-Phase Series RLC Branch/RConn3 -- Three-Phase Series RLC Branch2/LConn3 -- Three-Phase Series RLC Branch1/LConn3
  Three-Phase Series RLC Branch2/RConn2 -- Ground/LConn1 -- Three-Phase Series RLC Branch2/RConn3 -- Three-Phase Series RLC Branch2/RConn1
  Three-Phase V-I Measurement1/RConn1 -- Three-Phase Series RLC Branch/LConn1
  Three-Phase Series RLC Branch/LConn2 -- Three-Phase V-I Measurement1/RConn2
  Three-Phase Series RLC Branch/LConn3 -- Three-Phase V-I Measurement1/RConn3

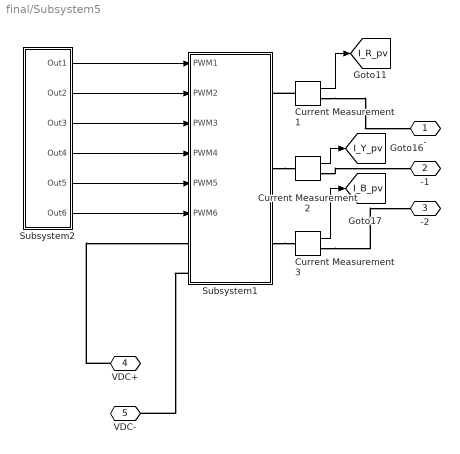
== system final/Subsystem5 ==
  Current Measurement1 : spsCurrentMeasurementLib/Current Measurement  PhasorSimulation=off  OutputType=Complex  PSBequivalent=0
  Current Measurement2 : spsCurrentMeasurementLib/Current Measurement  PhasorSimulation=off  OutputType=Complex  PSBequivalent=0
  Current Measurement3 : spsCurrentMeasurementLib/Current Measurement  PhasorSimulation=off  OutputType=Complex  PSBequivalent=0
  Subsystem1 : Subsystem
  Subsystem2 : Subsystem
  - : PMIOPort  Side=Right
  -1 : PMIOPort  Port=2  Side=Right
  -2 : PMIOPort  Port=3  Side=Right
  VDC+ : PMIOPort  Port=4  Side=Left
  VDC- : PMIOPort  Port=5  Side=Left
  tag scope: I_B_pv=global, I_R_pv=global, I_Y_pv=global
  wires:
  Current Measurement3/1 -> [I_B_pv]
  Subsystem2/3(Out3) -> Subsystem1/3(PWM3)
  Current Measurement1/1 -> [I_R_pv]
  Subsystem2/5(Out5) -> Subsystem1/5(PWM5)
  Subsystem2/2(Out2) -> Subsystem1/2(PWM2)
  Subsystem2/1(Out1) -> Subsystem1/1(PWM1)
  Subsystem2/6(Out6) -> Subsystem1/6(PWM6)
  Subsystem2/4(Out4) -> Subsystem1/4(PWM4)
  Current Measurement2/1 -> [I_Y_pv]
  connections:
  Subsystem1/RConn3 -- Current Measurement3/LConn1
  Subsystem1/RConn2 -- Current Measurement2/LConn1
  Current Measurement1/LConn1 -- Subsystem1/RConn1
  VDC+/RConn1 -- Subsystem1/LConn1
  Subsystem1/LConn2 -- VDC-/RConn1
  Current Measurement2/RConn1 -- -1/RConn1
  Current Measurement1/RConn1 -- -/RConn1
  Current Measurement3/RConn1 -- -2/RConn1

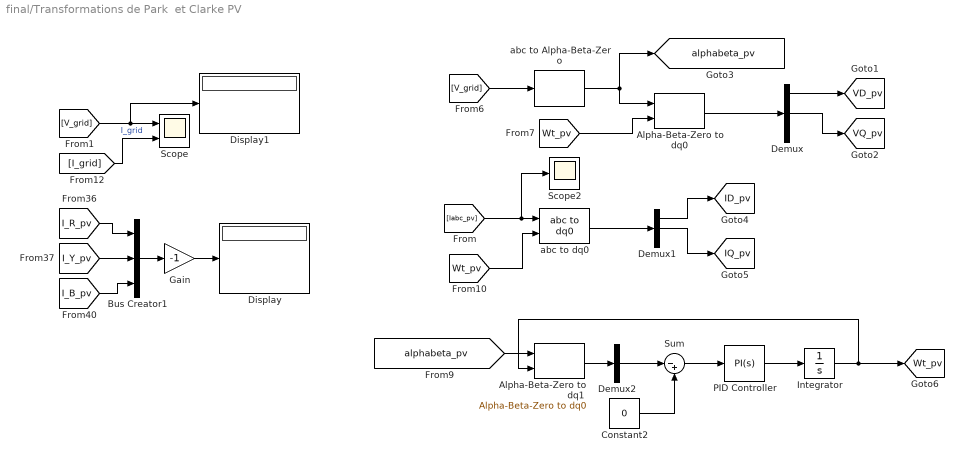
== system final/Transformations de Park  et Clarke PV ==
  Alpha-Beta-Zero to dq0 : spsAlphaBetaZerotodq0Lib/Alpha-Beta-Zero to dq0  Alignment=90 degrees behind phase A axis
  Alpha-Beta-Zero to dq1 : spsAlphaBetaZerotodq0Lib/Alpha-Beta-Zero to dq0  Alignment=90 degrees behind phase A axis
  Bus Creator1 : BusCreator  Inputs=3
  Constant2 : Constant  Value=0
  Demux : Demux  Outputs=3
  Demux1 : Demux  Outputs=3
  Demux2 : Demux  Outputs=3
  Display : Display
  Display1 : Display
  Gain : Gain  Gain=-1
  Integrator : Integrator
  PID Controller : slpidlib/PID Controller  Controller=PI  Form=Parallel  TimeDomain=Continuous-time  UseExternalTs=off  SampleTime=-1  IntegratorMethod=Forward Euler  FilterMethod=Forward Euler  ControllerParametersSource=internal  P=10  I=50000  UseKiTs=off  D=0  UseExternalDerivativeSource=off  N=100  UseFilter=on  TunerSelectOption=Transfer Function Based (PID Tuner App)  InitialConditionSource=internal  InitialConditionForIntegrator=0  InitialConditionForFilter=0  DifferentiatorICPrevScaledInput=0  ExternalReset=none  TrackingMode=off  Kt=1  LimitOutput=off  SatLimitsSource=internal  UpperSaturationLimit=inf  LowerSaturationLimit=-inf  LinearizeAsGain=on  AntiWindupMode=none  Kb=1  LimitIntegrator=off  UpperIntegratorSaturationLimit=inf  LowerIntegratorSaturationLimit=-inf  POutMin=[]  POutMax=[]  IOutMin=[]  IOutMax=[]  DOutMin=[]  DOutMax=[]  NOutMin=[]  NOutMax=[]  SumOutMin=[]  SumOutMax=[]  SaturationOutMin=[]  SaturationOutMax=[]  PParamMin=[]  PParamMax=[]  IParamMin=[]  IParamMax=[]  DParamMin=[]  DParamMax=[]  NParamMin=[]  NParamMax=[]  KbParamMin=[]  KbParamMax=[]  KtParamMin=[]  KtParamMax=[]  KbOutMin=[]  KbOutMax=[]  KtOutMin=[]  KtOutMax=[]  IntegratorOutMin=[]  IntegratorOutMax=[]  FilterOutMin=[]  FilterOutMax=[]  SumI1OutMin=[]  SumI1OutMax=[]  SumI2OutMin=[]  SumI2OutMax=[]  SumI3OutMin=[]  SumI3OutMax=[]  SumI4OutMin=[]  SumI4OutMax=[]  SumDOutMin=[]  SumDOutMax=[]  DifferentiatorOutMin=[]  DifferentiatorOutMax=[]  FilterDiffOutCoefMin=[]  FilterDiffOutCoefMax=[]  ReciprocalOutMin=[]  ReciprocalOutMax=[]  SumDenOutMin=[]  SumDenOutMax=[]  SumNumOutMin=[]  SumNumOutMax=[]  DivideOutMin=[]  DivideOutMax=[]  UdiffTsProdOutMin=[]  UdiffTsProdOutMax=[]  NTsProdOutMin=[]  NTsProdOutMax=[]  UintegralTsProdOutMin=[]  UintegralTsProdOutMax=[]  UngainTsProdOutMin=[]  UngainTsProdOutMax=[]  ClampingZeroOutDataTypeStr=Inherit: Inherit via back propagation  ClampingZeroOutMin=[]  ClampingZeroOutMax=[]  FilterDenConstantOutDataTypeStr=Inherit: Inherit via back propagation  FilterDenConstantOutMin=[]  FilterDenConstantOutMax=[]  PCopyOutDataTypeStr=Inherit: Inherit via back propagation  PCopyOutMin=[]  PCopyOutMax=[]  NCopyOutDataTypeStr=Inherit: Inherit via back propagation  NCopyOutMin=[]  NCopyOutMax=[]  IntegratorContinuousStateAttributes=''  IntegratorStateMustResolveToSignalObject=off  IntegratorRTWStateStorageClass=Auto  FilterContinuousStateAttributes=''  FilterStateMustResolveToSignalObject=off  FilterRTWStateStorageClass=Auto  ParallelPVariant=InternalParameters  IdealPVariant=Disabled  IVariant=InternalParameters  DVariant=Disabled  IntegratorVariant=Continuous  SatVariant=Disabled  AWVariant=Passthrough  PCopyVariant=Disabled  TRVariant=Disabled  FdbkBlocksVariant=Forward  IdealPFdbkVariant=Disabled  SatFdbkVariant=Disabled  DerivativeFilterVariant=Disabled  NVariant=Disabled  NCopyVariant=Disabled_SignalSpec  FilterICVariant=Disabled  IntegratorICVariant=InternalICs  ExternalResetVariant=Disabled  TRSumVariant=Passthrough  SumFdbkVariant=Disabled  SumVariant=Sum_PI  TsampFilterVariant=InternalTs  TsampNgainVariant=Passthrough  TsampIntegralVariant=Disabled_SignalSpec  ExternalSaturationOutDataTypeStr=Inherit: Same as second input  DerivativeSourceVariant=Disabled
  Scope : Scope  NumInputPorts=2
  Scope2 : Scope
  Sum : Sum  Inputs=|-+
  abc to Alpha-Beta-Zero : spsabctoAlphaBetaZeroLib/abc to Alpha-Beta-Zero
  abc to dq0 : spsabctodq0Lib/abc to dq0  Alignment=90 degrees behind phase A axis
  tag scope: ID_pv=global, IQ_pv=global, VD_pv=global, VQ_pv=global, Wt_pv=global, alphabeta_pv=global
  wires:
  Integrator/1 -> [Wt_pv], Alpha-Beta-Zero to dq1/2
  abc to Alpha-Beta-Zero/1 -> Alpha-Beta-Zero to dq0/1, [alphabeta_pv]
  Demux1/1 -> [ID_pv]
  Sum/1 -> PID Controller/1
  Demux/1 -> [VD_pv]
  Demux1/2 -> [IQ_pv]
  PID Controller/1 -> Integrator/1
  abc to dq0/1 -> Demux1/1
  Constant2/1 -> Sum/2
  [V_grid] -> abc to Alpha-Beta-Zero/1
  [Wt_pv] -> Alpha-Beta-Zero to dq0/2
  Alpha-Beta-Zero to dq0/1 -> Demux/1
  Alpha-Beta-Zero to dq1/1 -> Demux2/1
  [alphabeta_pv] -> Alpha-Beta-Zero to dq1/1
  Demux/2 -> [VQ_pv]
  Demux2/2 -> Sum/1
  [Wt_pv] -> abc to dq0/2
  Bus Creator1/1 -> Gain/1
  [I_B_pv] -> Bus Creator1/3
  [I_R_pv] -> Bus Creator1/1
  [I_Y_pv] -> Bus Creator1/2
  Gain/1 -> Display/1
  [V_grid] -> Display1/1, Scope/1
  [I_grid] -> Scope/2  "I_grid"
  [Iabc_pv] -> Scope2/1, abc to dq0/1

== system final/Charge Variable/Dynamic Load Control ==
  P0 : Inport
  Fcn : Fcn  Expr=sqrt(1/u(1)^2-1)
  Mux : Mux  Inputs=2
  Product : Product
  Summer1 : Constant  Value=PF
  PQ : Outport  VectorParamsAs1DForOutWhenUnconnected=off
  wires:
  Summer1/1 -> Fcn/1
  Fcn/1 -> Product/2
  P0/1 -> Product/1, Mux/1
  Mux/1 -> PQ/1
  Product/1 -> Mux/2  "Qo"

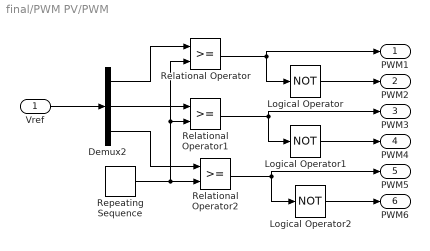
== system final/PWM PV/PWM ==
  Vref : Inport
  Demux2 : Demux  Outputs=3
  Logical Operator : Logic  Operator=NOT  AllPortsSameDT=off  OutDataTypeStr=boolean
  Logical Operator1 : Logic  Operator=NOT  AllPortsSameDT=off  OutDataTypeStr=boolean
  Logical Operator2 : Logic  Operator=NOT  AllPortsSameDT=off  OutDataTypeStr=boolean
  Relational Operator : RelationalOperator  OutDataTypeStr=boolean  RndMeth=Simplest  InputSameDT=off
  Relational Operator1 : RelationalOperator  OutDataTypeStr=boolean  RndMeth=Simplest  InputSameDT=off
  Relational Operator2 : RelationalOperator  OutDataTypeStr=boolean  RndMeth=Simplest  InputSameDT=off
  Repeating Sequence : simulink/Sources/Repeating Sequence  rep_seq_t=[0 0.00005 0.0001]  rep_seq_y=[-1 1 -1]
  PWM1 : Outport
  PWM2 : Outport  Port=2
  PWM3 : Outport  Port=3
  PWM4 : Outport  Port=4
  PWM5 : Outport  Port=5
  PWM6 : Outport  Port=6
  wires:
  Logical Operator/1 -> PWM2/1
  Logical Operator2/1 -> PWM6/1
  Vref/1 -> Demux2/1
  Relational Operator2/1 -> PWM5/1, Logical Operator2/1
  Logical Operator1/1 -> PWM4/1
  Repeating Sequence/1 -> Relational Operator2/2, Relational Operator1/2, Relational Operator/2
  Relational Operator/1 -> PWM1/1, Logical Operator/1
  Relational Operator1/1 -> PWM3/1, Logical Operator1/1
  Demux2/1 -> Relational Operator/1
  Demux2/3 -> Relational Operator2/1
  Demux2/2 -> Relational Operator1/1

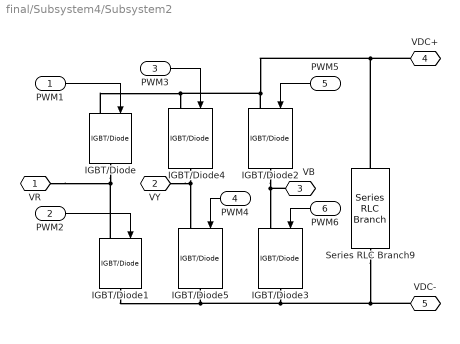
== system final/Subsystem4/Subsystem2 ==
  "PWM1 " : Inport
  PWM2 : Inport  Port=2
  PWM3 : Inport  Port=3
  PWM4 : Inport  Port=4
  PWM5 : Inport  Port=5
  PWM6 : Inport  Port=6
  IGBT/Diode{,1..5} (6 alike) : spsIGBTDiodeLib/IGBT//Diode  Ron=1e-3  Rs=1e5  Cs=inf  Measurements=off
  Series RLC Branch9 : spsSeriesRLCBranchLib/Series RLC Branch  LConnTagsString=__new0  RConnTagsString=__new0  BranchType=RC  Resistance=3291e-4  Inductance=1e-3  SetiL0=off  InitialCurrent=0  Capacitance=63e-4  Setx0=on  InitialVoltage=800  Measurements=None
  VR : PMIOPort  Side=Left
  VY : PMIOPort  Port=2  Side=Left
  VB : PMIOPort  Port=3  Side=Left
  VDC+ : PMIOPort  Port=4  Side=Right
  VDC- : PMIOPort  Port=5  Side=Right
  wires:
  PWM3/1 -> IGBT/Diode4/1
  PWM6/1 -> IGBT/Diode3/1
  PWM5/1 -> IGBT/Diode2/1
  PWM2/1 -> IGBT/Diode1/1
  "PWM1 "/1 -> IGBT/Diode/1
  PWM4/1 -> IGBT/Diode5/1
  connections:
  VR/RConn1 -- IGBT/Diode1/LConn1 -- IGBT/Diode/RConn1
  Series RLC Branch9/RConn1 -- VDC-/RConn1 -- IGBT/Diode3/RConn1 -- IGBT/Diode1/RConn1 -- IGBT/Diode5/RConn1
  IGBT/Diode4/RConn1 -- VY/RConn1 -- IGBT/Diode5/LConn1
  Series RLC Branch9/LConn1 -- VDC+/RConn1 -- IGBT/Diode/LConn1 -- IGBT/Diode4/LConn1 -- IGBT/Diode2/LConn1
  IGBT/Diode2/RConn1 -- VB/RConn1 -- IGBT/Diode3/LConn1

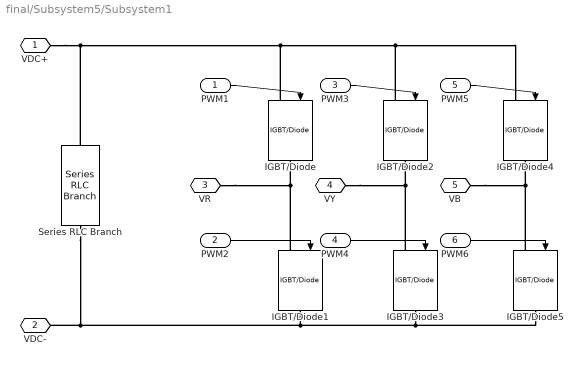
== system final/Subsystem5/Subsystem1 ==
  PWM1 : Inport
  PWM2 : Inport  Port=2
  PWM3 : Inport  Port=3
  PWM4 : Inport  Port=4
  PWM5 : Inport  Port=5
  PWM6 : Inport  Port=6
  IGBT/Diode{,1..5} (6 alike) : spsIGBTDiodeLib/IGBT//Diode  Ron=1e-3  Rs=1e5  Cs=inf  Measurements=off
  Series RLC Branch : spsSeriesRLCBranchLib/Series RLC Branch  LConnTagsString=__new0  RConnTagsString=__new0  BranchType=RC  Resistance=1e-3  Inductance=1e-3  SetiL0=off  InitialCurrent=0  Capacitance=5600e-6  Setx0=off  InitialVoltage=800  Measurements=None
  VDC+ : PMIOPort  Side=Left
  VDC- : PMIOPort  Port=2  Side=Left
  VR : PMIOPort  Port=3  Side=Right
  VY : PMIOPort  Port=4  Side=Right
  VB : PMIOPort  Port=5  Side=Right
  wires:
  PWM2/1 -> IGBT/Diode1/1
  PWM5/1 -> IGBT/Diode4/1
  PWM3/1 -> IGBT/Diode2/1
  PWM1/1 -> IGBT/Diode/1
  PWM4/1 -> IGBT/Diode3/1
  PWM6/1 -> IGBT/Diode5/1
  connections:
  IGBT/Diode3/LConn1 -- VY/RConn1 -- IGBT/Diode2/RConn1
  IGBT/Diode1/LConn1 -- VR/RConn1 -- IGBT/Diode/RConn1
  VDC+/RConn1 -- IGBT/Diode/LConn1 -- IGBT/Diode2/LConn1 -- IGBT/Diode4/LConn1 -- Series RLC Branch/LConn1
  IGBT/Diode5/LConn1 -- VB/RConn1 -- IGBT/Diode4/RConn1
  IGBT/Diode5/RConn1 -- IGBT/Diode3/RConn1 -- Series RLC Branch/RConn1 -- VDC-/RConn1 -- IGBT/Diode1/RConn1

== system final/Subsystem5/Subsystem2 ==
  Out1 : Outport
  Out2 : Outport  Port=2
  Out3 : Outport  Port=3
  Out4 : Outport  Port=4
  Out5 : Outport  Port=5
  Out6 : Outport  Port=6
  wires:
  [PMW3] -> Out3/1
  [PMW2] -> Out2/1
  [PMW4] -> Out4/1
  [PMW5] -> Out5/1
  [PMW6] -> Out6/1
  [PMW1] -> Out1/1

== matlab function final/Subsystem/MATLAB Function ==
  data: V input; Vref output; I input
function Vref = RefGen(V, I)
% Générateur de référence de tension MPPT (Perturb & Observe)
% V : tension PV (V)
% I : courant PV (A)
% Vref : référence de tension (V)

% --- Limites et initialisation (à adapter à ton string) ---
Vrefmin  = 0.0;
Vrefmax  = 330;     % proche de Voc
Vrefinit = 290;     % proche de Vmpp string (ordre de grandeur)
deltaVref = 1;      % pas de perturbation (V)

% --- Seuils anti-bruit (à ajuster) ---
epsP = 5;           % W : zone morte sur la puissance
epsV = 0.2;         % V : zone morte sur la tension

persistent Vold Pold Vrefold
if isempty(Vold)
    Vold = V;
    Pold = V*I;
    Vrefold = Vrefinit;
end

% --- Calculs ---
P  = V*I;
dV = V - Vold;
dP = P - Pold;

% --- Anti-bruit : si variations trop faibles, on garde Vref ---
if abs(dP) < epsP || abs(dV) < epsV
    Vref = Vrefold;
else
    % --- P&O classique (même logique que ton code) ---
    if dP < 0
        if dV < 0
            Vref = Vrefold + deltaVref;
        else
            Vref = Vrefold - deltaVref;
        end
    else
        if dV < 0
            Vref = Vrefold - deltaVref;
        else
            Vref = Vrefold + deltaVref;
        end
    end
end

% --- Saturation ---
if (Vref >= Vrefmax) || (Vref <= Vrefmin)
    Vref = Vrefold;
end

% --- Mise à jour des mémoires ---
Vrefold = Vref;
Vold = V;
Pold = P;
end

== stateflow chart final/Chart ==
  state Systeme_de_gestion_d_energie
    during : P_net = P_pv - P_load;
    state ACHAT_RESEAU
      entry : P_bat_ref = 0; mode = 4; P_grid = 0;
      during : P_pv_ref = min(P_pv, P_load); % 1) Puissance PV utilisée pour la charge
      P_deficit = P_load - P_pv_ref; % 2) Déficit de puissance
      % 3) Gestion batterie
      if SOC < SOC_min
      % Batterie protégée → recharge obligatoire
      P_bat_ref = P_ch_max;     % charge batterie (positive)
      elseif SOC < SOC_max
      % Batterie normale → recharge possible
      P_bat_ref = min(P_ch_max, P_grid_max);
      else
      % Batterie pleine
      P_bat_ref = 0;
      end
      % 4) Puissance réseau = charge + recharge batterie
      P_grid = P_deficit + P_bat_ref;
    state CHARGE_ET_VENTE_RESEAU
      entry: mode = 6;
      P_grid = 0;
      P_bat_ref = 0;
      during : % PV alimente la charge en priorité
      P_pv_ref = min(P_pv, P_load);
      % surplus PV
      P_surplus = P_pv - P_pv_ref;
      % 1) Charge batterie si possible
      if SOC < SOC_max
      P_bat_ref = min(P_surplus, P_ch_max);    % positif = charge
      else
      P_bat_ref = 0;
      end
      % 2) Vendre le surplus restant au réseau (si réseau disponible)
      if grid_on == 1
      P_restant = P_surplus - P_bat_ref;       % ce qui reste après charge batt
      if P_restant > 0
      P_grid = -P_restant;                 % négatif = vente (export)
      else
      P_grid = 0;
      end
      else
      P_grid = 0;   % réseau coupé => pas de vente
      end
    state PV_ALIMENTE_CHARGE
      entry:
      P_bat_ref = 0;
      P_grid = 0;
      during : mode =1;
      P_pv_ref = min(P_pv, P_load);
    state CHARGE_BATTERIE_vente_surplus
      entry:
      P_grid = 0;
      during: mode =2;
      P_pv_ref = min(P_pv, P_load);
      P_surplus = P_pv - P_pv_ref;
      P_bat_ref = min(P_surplus, P_ch_max);
      P_grid =  -(P_pv-P_pv_ref-P_bat_ref);
    state DECHARGE_BATTERIE
      entry: mode = 3;
      P_grid = 0;
      P_bat_ref = 0;
      during:
      % 1) Puissance PV réellement utilisée
      P_pv_ref = min(P_pv, P_load);
      % 2) Déficit de puissance
      P_deficit = P_load - P_pv_ref;
      % 3) Protection SOC : ne pas décharger si batterie trop basse
      if SOC <= SOC_min
      P_bat_ref = 0;
      else
      % Décharge batterie (puissance négative)
      P_bat_ref = -min(P_deficit, P_dis_max);
      end
      % 4) Gestion du réseau
      if grid_on == 1
      % Le réseau fournit ce que la batterie ne peut pas fournir
      P_grid = P_deficit - (-P_bat_ref);
      else
      % Réseau coupé
      P_grid = 0;
      end
    state VENTE_SEULE
      entry: mode = 7;
      P_bat_ref = 0;
      P_grid = 0;
      during: P_pv_ref = min(P_pv, P_load);
      P_surplus = P_pv - P_pv_ref;
      % Batterie pleine => pas de charge
      P_bat_ref = 0;
      % Vendre tout le surplus
      if grid_on == 1 && P_surplus > 0
      P_grid = -P_surplus;
      else
      P_grid = 0;
      end
    state MODE_ILOTAGE
      entry : P_grid = 0; mode = 5;
      during : P_pv_ref = min(P_pv, P_load);
      P_deficit = P_load - P_pv_ref;
      if SOC > SOC_min
      P_bat_ref = -min(P_deficit, P_dis_max);
      P_non_alimente = max(0, P_deficit - (-P_bat_ref));
      else
      P_bat_ref = 0;
      P_non_alimente = P_deficit;
      end
    note: Convention des puissances (signes)
    note: P_pv​≥0 : puissance PV disponible
        | P_pv_ref≥0 : puissance PV réellement utilisée
        | (vers charge + éventuellement batterie)
    note: Pgrid​>0 : achat / import depuis le réseau
        | Pgrid<0 : vente / export vers le réseau
        | Pgrid=0 : réseau non utilisé / coupé
    note: P_bat_ref​>0 : charge de la batterie
        | P_bat_ref<0 : décharge de la batterie
        | P_bat_ref=0 : batterie neutre
    (default) -> PV_ALIMENTE_CHARGE
    ACHAT_RESEAU -> DECHARGE_BATTERIE [order 3] : [SOC > SOC_min + 2 && P_net < -epsP]
    ACHAT_RESEAU -> PV_ALIMENTE_CHARGE [order 1] : [P_net >= -epsP]
    PV_ALIMENTE_CHARGE -> ACHAT_RESEAU [order 4] : [P_net < -epsP && SOC <= SOC_min]
    ACHAT_RESEAU -> MODE_ILOTAGE [order 4] : [grid_on == 0]
    CHARGE_BATTERIE_vente_surplus -> ACHAT_RESEAU [order 3] : [P_net < -epsP && SOC <= SOC_min]
    ACHAT_RESEAU -> CHARGE_BATTERIE_vente_surplus [order 2] : [P_net > epsP && SOC < SOC_max]
    CHARGE_BATTERIE_vente_surplus -> CHARGE_ET_VENTE_RESEAU [order 4] : [grid_on==1 && (P_pv - min(P_pv,P_load)) > P_ch_max && SOC < SOC_max]
    PV_ALIMENTE_CHARGE -> CHARGE_BATTERIE_vente_surplus [order 1] : [P_net > epsP && SOC < SOC_max]
    CHARGE_BATTERIE_vente_surplus -> PV_ALIMENTE_CHARGE [order 1] : [P_net <= epsP || SOC >= SOC_max]
    CHARGE_ET_VENTE_RESEAU -> CHARGE_BATTERIE_vente_surplus [order 1] : [(P_pv - min(P_pv,P_load)) <= P_ch_max || grid_on==0]
    CHARGE_BATTERIE_vente_surplus -> DECHARGE_BATTERIE [order 2] : [P_net < -epsP && SOC > SOC_min]
    MODE_ILOTAGE -> CHARGE_BATTERIE_vente_surplus [order 1] : [grid_on == 1 && P_net > epsP && SOC < SOC_max]
    CHARGE_ET_VENTE_RESEAU -> PV_ALIMENTE_CHARGE [order 2] : [P_net <= epsP]
    PV_ALIMENTE_CHARGE -> CHARGE_ET_VENTE_RESEAU [order 5] : [grid_on==1 && P_net > epsP && SOC < SOC_max]
    DECHARGE_BATTERIE -> PV_ALIMENTE_CHARGE [order 1] : [P_net >= -epsP]
    PV_ALIMENTE_CHARGE -> DECHARGE_BATTERIE [order 3] : [P_net < -epsP && SOC > SOC_min]
    MODE_ILOTAGE -> PV_ALIMENTE_CHARGE [order 3] : [grid_on == 1]
    PV_ALIMENTE_CHARGE -> MODE_ILOTAGE [order 2] : [grid_on == 0]
    VENTE_SEULE -> PV_ALIMENTE_CHARGE [order 1] : [P_net <= epsP]
    PV_ALIMENTE_CHARGE -> VENTE_SEULE [order 6] : [grid_on==1 && P_net > epsP && SOC >= SOC_max]
    VENTE_SEULE -> CHARGE_ET_VENTE_RESEAU [order 2] : [SOC < SOC_max && P_net > epsP && grid_on==1]
    CHARGE_ET_VENTE_RESEAU -> VENTE_SEULE [order 3] : [SOC >= SOC_max && P_net > epsP && grid_on==1]
    MODE_ILOTAGE -> DECHARGE_BATTERIE [order 2] : [grid_on == 1 && P_net < -epsP && SOC > SOC_min]
    DECHARGE_BATTERIE -> MODE_ILOTAGE [order 2] : [SOC <= SOC_min && ~grid_on]
  (default) -> Systeme_de_gestion_d_energie : {P_net = P_pv - P_load;} % Puissance nette (pour transitions)
  data: P_pv input; P_load input; P_pv_ref output; P_bat_ref output; P_grid output; P_net output; P_ch_max local =5; P_surplus local; epsP constant double =0.5; SOC input; SOC_max constant double =90; mode output; grid_on input; P_dis_max local =5; P_deficit local; SOC_min constant double =20; P_non_alimente output; P_restant output; P_grid_max constant double =10
